simulink model "WaterTankSysControl2018"  (R2015b)
settings: Solver=FixedStepAuto  StartTime=0.0  StopTime=5*140*0.75  FixedStep=0.75  RelTol=1e-3
undefined symbols (not defined in the file or in its folder): MIO, National_Instruments, PCI
libraries: sldrtlib x4, simulink x1
settings Model: SimulationMode=external  ExtModeTrigDuration=7200  ExtModeArchiveMode=auto  ExtModeArchiveFileName=SFControlData  ExtModeArchiveDirName=C:\Users\My Project\Documents\MATLAB  ExtModeAutoIncOneShot=on  ExtModeWriteAllDataToWs=on  Creator=My Project  LastModifiedBy=My Project
settings HardwareCC: ProdBitPerLong=64  ProdLargestAtomicFloat=None  ProdHWDeviceType=Intel->x86-64  TargetBitPerLong=64  TargetBitPerPointer=64  TargetIntDivRoundTo=Zero  TargetEndianess=LittleEndian  TargetWordSize=64  TargetHWDeviceType=Intel->x86-64
settings RTWCC: SystemTargetFile=sldrt.tlc  TemplateMakefile=sldrt.tmf  Description=Simulink Desktop Real-Time  RTWCompilerOptimization=on
settings CodeAppCC: MaxIdLength=95
settings SimulinkDesktopRealTimeCC: TargetPreCompLibLocation=C:\Program Files\MATLAB\R2015b\toolbox\sldrt\lib\win64  TargetLangStandard=C89/C90 (ANSI)  SupportVariableSizeSignals=off

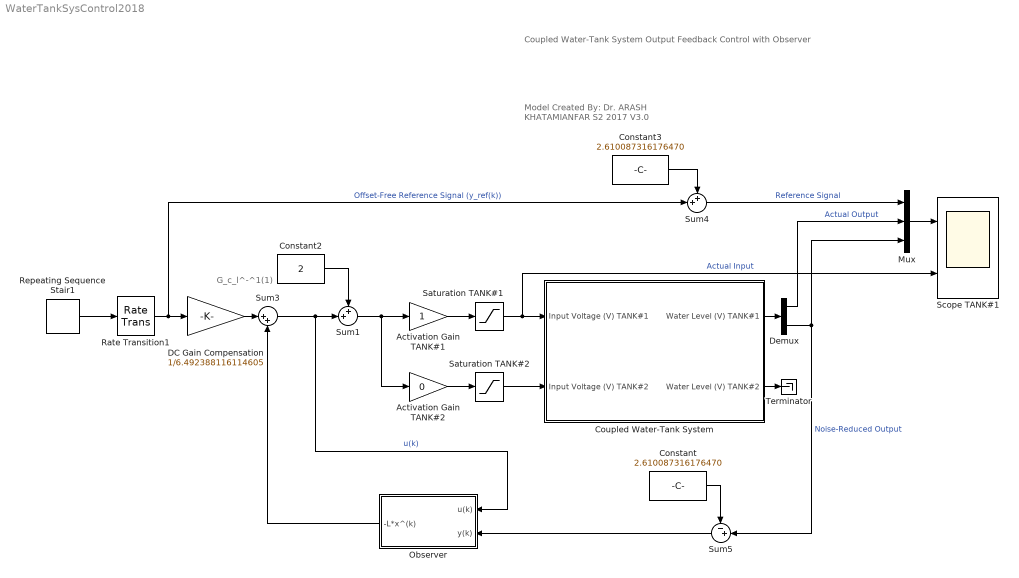
== system WaterTankSysControl2018 ==
  note: Model Created By:
      | Dr. ARASH KHATAMIANFAR
      | S2 2017 V3.0
  note: G_c_l^-^1(1)
  note: Coupled Water-Tank System
      | Output Feedback Control with Observer
  Activation Gain TANK#1 : Gain
  Activation Gain TANK#2 : Gain  Gain=0
  Constant : Constant  Value=2.610087316176470
  Constant2 : Constant  Value=2
  Constant3 : Constant  Value=2.610087316176470
  Coupled Water-Tank System : Subsystem
  DC Gain Compensation : Gain  Gain=1/6.492388116114605
  Demux : Demux  Outputs=2
  Mux : Mux  Inputs=3
  Observer : Subsystem
  Rate Transition1 : RateTransition  OutPortSampleTime=0.75
  Repeating Sequence Stair1 : simulink/Sources/Repeating Sequence Stair  OutValues=[0.7 0.2 -0.5 0].'  tsamp=140*0.75  OutMin=[]  OutMax=[]  OutDataTypeStr=double  OutputDataTypeScalingMode=double  OutDataType=fixdt(0,8)  ConRadixGroup=Best Precision: Vector-wise  OutScaling=2^-12
  Saturation TANK#1 : Saturate  UpperLimit=2.5  LowerLimit=1.5
  Saturation TANK#2 : Saturate  UpperLimit=5  LowerLimit=0
  Scope TANK#1 : Scope  NumInputPorts=2
  Sum1 : Sum  Inputs=++|
  Sum3 : Sum  Inputs=|++
  Sum4 : Sum  Inputs=++|
  Sum5 : Sum  Inputs=-+|
  Terminator : Terminator
  wires:
  Activation Gain TANK#1/1 -> Saturation TANK#1/1
  Activation Gain TANK#2/1 -> Saturation TANK#2/1
  Saturation TANK#2/1 -> Coupled Water-Tank System/2(Input Voltage (V) TANK#2)
  Sum1/1 -> Activation Gain TANK#2/1, Activation Gain TANK#1/1
  Coupled Water-Tank System/2(Water Level (V) TANK#2) -> Terminator/1
  Constant2/1 -> Sum1/1
  Sum3/1 -> Observer/1(u(k)), Sum1/2  "u(k)"
  DC Gain Compensation/1 -> Sum3/1
  Observer/1(-L*x^(k)) -> Sum3/2
  Sum5/1 -> Observer/2(y(k))
  Constant/1 -> Sum5/1
  Rate Transition1/1 -> Sum4/2, DC Gain Compensation/1  "Offset-Free Reference Signal (y_ref(k))"
  Repeating Sequence Stair1/1 -> Rate Transition1/1
  Constant3/1 -> Sum4/1
  Sum4/1 -> Mux/1  "Reference Signal"
  Mux/1 -> Scope TANK#1/1
  Saturation TANK#1/1 -> Coupled Water-Tank System/1(Input Voltage (V) TANK#1), Scope TANK#1/2  "Actual Input"
  Coupled Water-Tank System/1(Water Level (V) TANK#1) -> Demux/1
  Demux/1 -> Mux/2  "Actual Output"
  Demux/2 -> Sum5/2, Mux/3  "Noise-Reduced Output"

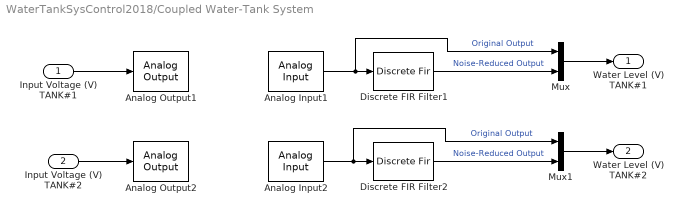
== system WaterTankSysControl2018/Coupled Water-Tank System ==
  Input Voltage (V) TANK#1 : Inport
  Input Voltage (V) TANK#2 : Inport  Port=2
  Analog Input1 : sldrtlib/Analog Input  SampleTime=0.75  MaxMissedTicks=10  ShowMissedTicks=off  YieldWhenWaiting=off  DrvName=National_Instruments/PCI-MIO-16E-4  DrvAddress=4294967295  DrvOptions=[0 0 0 0 0 0]  Channels=1  RangeMode=1  VoltRange=1  DataType=1
      settings: AttributesFormatString=National Instruments\nPCI-MIO-16E-4 [auto]
  Analog Input2 : sldrtlib/Analog Input  SampleTime=0.75  MaxMissedTicks=10  ShowMissedTicks=off  YieldWhenWaiting=off  DrvName=National_Instruments/PCI-MIO-16E-4  DrvAddress=4294967295  DrvOptions=[0 0 0 0 0 0]  Channels=2  RangeMode=1  VoltRange=1  DataType=1
      settings: AttributesFormatString=National Instruments\nPCI-MIO-16E-4 [auto]
  Analog Output1 : sldrtlib/Analog Output  SampleTime=0.75  MaxMissedTicks=10  ShowMissedTicks=off  YieldWhenWaiting=off  DrvName=National_Instruments/PCI-MIO-16E-4  DrvAddress=4294967295  DrvOptions=[0 0 0 0 0 0]  Channels=1  RangeMode=1  VoltRange=1  InitialValue=0  FinalValue=0
      settings: AttributesFormatString=National Instruments\nPCI-MIO-16E-4 [auto]
  Analog Output2 : sldrtlib/Analog Output  SampleTime=0.75  MaxMissedTicks=10  ShowMissedTicks=off  YieldWhenWaiting=off  DrvName=National_Instruments/PCI-MIO-16E-4  DrvAddress=4294967295  DrvOptions=[0 0 0 0 0 0]  Channels=2  RangeMode=1  VoltRange=1  InitialValue=0  FinalValue=0
      settings: AttributesFormatString=National Instruments\nPCI-MIO-16E-4 [auto]
  Discrete FIR Filter1 : DiscreteFir  Coefficients=[0.2 0.2 0.2 0.2 0.2]  SampleTime=0.75
  Discrete FIR Filter2 : DiscreteFir  Coefficients=[0.2 0.2 0.2 0.2 0.2]  SampleTime=0.75
  Mux : Mux  Inputs=2
  Mux1 : Mux  Inputs=2
  Water Level (V) TANK#1 : Outport
  Water Level (V) TANK#2 : Outport  Port=2
  wires:
  Analog Input1/1 -> Mux/1, Discrete FIR Filter1/1  "Original Output"
  Input Voltage (V) TANK#1/1 -> Analog Output1/1
  Discrete FIR Filter1/1 -> Mux/2  "Noise-Reduced Output"
  Mux/1 -> Water Level (V) TANK#1/1
  Analog Input2/1 -> Mux1/1, Discrete FIR Filter2/1  "Original Output"
  Input Voltage (V) TANK#2/1 -> Analog Output2/1
  Discrete FIR Filter2/1 -> Mux1/2  "Noise-Reduced Output"
  Mux1/1 -> Water Level (V) TANK#2/1

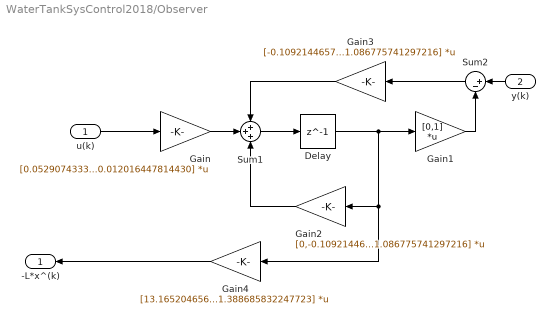
== system WaterTankSysControl2018/Observer ==
  u(k) : Inport
  y(k) : Inport  Port=2
  Delay : Delay  DelayLength=1  InitialCondition=[0;0]  SampleTime=0.75
  Gain : Gain  Gain=[0.052907433346716;0.012016447814430]  Multiplication=Matrix(K*u)
  Gain1 : Gain  Gain=[0,1]  Multiplication=Matrix(K*u)
  Gain2 : Gain  Gain=[0,-0.109214465733547;1,1.086775741297216]  Multiplication=Matrix(K*u)
  Gain3 : Gain  Gain=[-0.109214465733547;1.086775741297216]  Multiplication=Matrix(K*u)
  Gain4 : Gain  Gain=[13.165204656675620,1.388685832247723]  Multiplication=Matrix(K*u)
  Sum1 : Sum  Inputs=+++
  Sum2 : Sum  Inputs=|+-
  -L*x^(k) : Outport
  wires:
  Delay/1 -> Gain1/1, Gain4/1, Gain2/1
  Sum2/1 -> Gain3/1
  Sum1/1 -> Delay/1
  Gain/1 -> Sum1/2
  Gain1/1 -> Sum2/2
  Gain2/1 -> Sum1/3
  Gain3/1 -> Sum1/1
  y(k)/1 -> Sum2/1
  u(k)/1 -> Gain/1
  Gain4/1 -> -L*x^(k)/1
